simulink model "SimplifiedModelWithRefSearch"  (R2022b)
settings: Solver=VariableStepAuto  StartTime=0.0  StopTime=inf  RelTol=1e-3
model workspace (MAT data in the model file):
  firstWarning = 1
  originalScenarioChecksum = '114339432DE22364D47BB28FC96DC10C'
undefined symbols (not defined in the file): Acceleration, ActorID, AngularVelocity, curvature1, DefaultGear, DEND_B, DEND_S, DEND_T, EgoRefPose, LF, LR, MAX_BRAKE, MAX_STEER, MAX_TORQUE, MCAR, MIN_BRAKE, MIN_STEER, MIN_TORQUE, NUMD_B, NUMD_S, NUMD_T, Pitch, Position, psi_o, R, Roll, RRdamp, session, sigbuilder_block, STEER_RATIO, stopSign_ID, Tdead, TL_ID, TrackWidth, ts, Ts, Vdead, Velocity, X_o, Y_o, Yaw
libraries: drivingvehiclecontroller x2, drivingscenarioandsensors x2, autolibshared x1, vehdynlibviscommon x1, vehdynlibsteering x1
(part 2 of 2)

== matlab function SimplifiedModelWithRefSearch/MATLAB Function ==
  data: RefPose input; RPose output; CurPose input; Curvature output; RefCurve input; j output
function [RPose,Curvature,j] = RefPoseSearch(RefPose,CurPose, RefCurve)

RPose = zeros(1,3);
% RPose = CurPose;
Curvature = 0;
%br = 0;
m = 0; mm = 0; b = 0; bb = 0;
% dth =  5;
% RefPose(:,2:3) = -RefPose(:,2:3);
% CurPose(2:3) = -CurPose(2:3);
dist = zeros(length(RefPose),1);
% a1 =0;a2 =0;a3 =0;a4 =0;

for j = 1:length(RefPose)
    dist(j) = norm(CurPose(1:2) - RefPose(j,1:2));
end

[val,ind] = mink(dist,2);
j = ind(1);

if ind(1) > ind(2)
    ind = [ind(2) ;ind(1)];
end
    
m = (RefPose(ind(1),2) - RefPose(ind(2),2))/(RefPose(ind(1),1) - RefPose(ind(2),1));
if m == inf
    RPose = [RefPose(ind(1),1) CurPose(2) atan2d(RefPose(ind(2),2)-RefPose(ind(2),2),RefPose(ind(2),1)-RefPose(ind(2),1))];
elseif m == 0
    RPose = [CurPose(1) RefPose(ind(1),2) atan2d(RefPose(ind(2),2)-RefPose(ind(2),2),RefPose(ind(2),1)-RefPose(ind(2),1))];
else
    b = RefPose(ind(1),2) - m*RefPose(ind(1),1);
    mm = -1/m;
    bb = CurPose(2) - mm*CurPose(1);
    RPose(1:2) = [(b-bb)/(mm-m) m*((b-bb)/(mm-m))+b]; 
%     RPose(3) = atan2d(-(RefPose(ind(1),2)-RPose(2)),-(RefPose(ind(1),1)-RPose(1))); % RefPose(ind(1),3);
    Curvature = RefCurve(ind(1));
     RPose(3) = RefPose(ind(1),3);

%     RPose(3) = (RefPose(ind(1),3) + RefPose(ind(2),3))/2;
%     Curvature = (RefCurve(ind(1)) + RefCurve(ind(2)))/2;

%     if abs(RefPose(ind(1),3)) < 45 || abs(RefPose(ind(1),3)) > 135
%         Curvature = interp1([RefPose(ind(1),1) RefPose(ind(2),1)],[RefCurve(ind(1)) RefCurve(ind(2))],CurPose(1));
%         RPose(3) = interp1([RefPose(ind(1),1) RefPose(ind(2),1)],[RefPose(ind(1),3) RefPose(ind(2),3)],CurPose(1));
%     else
% %         a1 =RefPose(ind(1),2);a2 =RefPose(ind(2),2);a3 =RefPose(ind(1),3);a4 =RefPose(ind(2),3);
%         Curvature = interp1([RefPose(ind(1),2) RefPose(ind(2),2)],[RefCurve(ind(1)) RefCurve(ind(2))],CurPose(2));
%         RPose(3) = interp1([RefPose(ind(1),2) RefPose(ind(2),2)],[RefPose(ind(1),3) RefPose(ind(2),3)],CurPose(2));
%     end
end



% for j = 1:length(RefPose)-1
%     
%     if (CurPose(3) >= -90 && CurPose(3) <= 90) % Ego vehicle is heading to the "right"
% 
%         if (RefPose(j,3) >= 0 && RefPose(j,3) <= 90) % Positive slope path
%             if RefPose(j,3) > dth && RefPose(j,3) < 90-dth % Ref path is not horizontal nor vertical
% 
%                 if (CurPose(1) >= RefPose(j,1) && CurPose(1) < RefPose(j+1,1)) && (CurPose(2) >= RefPose(j,2) && CurPose(2) < RefPose(j+1,2))
%                     m = (RefPose(j+1,2) - RefPose(j,2))/(RefPose(j+1,1) - RefPose(j,1));
%                     if m == inf
%                         RPose = [RefPose(j,1) CurPose(2) atan2d(RefPose(j+1,2)-RefPose(j,2),RefPose(j+1,1)-RefPose(j,1))];
%                     elseif m == 0
%                         RPose = [CurPose(1) RefPose(j,2) atan2d(RefPose(j+1,2)-RefPose(j,2),RefPose(j+1,1)-RefPose(j,1))];
%                     else
%                         b = RefPose(j,2) - m*RefPose(j,1);
%                         mm = -1/m;
%                         bb = CurPose(2) - mm*CurPose(1);
%                         RPose(1:2) = [(b-bb)/(mm-m) m*((b-bb)/(mm-m))+b];
%                         RPose(3) = interp1([RefPose(j,1) RefPose(j+1,1)],[RefPose(j,3) RefPose(j+1,3)],CurPose(1)); % or atan2d
%                         Curvature = interp1([RefPose(j,1) RefPose(j+1,1)],[RefCurve(j) RefCurve(j+1)],CurPose(1));
%                     end
%                     break;
%                 else
%                     continue
%                 end
% 
%             elseif RefPose(j,3) < dth % Ref path is horizontal
%                 if (CurPose(1) >= RefPose(j,1) && CurPose(1) < RefPose(j+1,1))
%                     m = (RefPose(j+1,2) - RefPose(j,2))/(RefPose(j+1,1) - RefPose(j,1));
%                     if m == inf
%                         RPose = [RefPose(j,1) CurPose(2) atan2d(RefPose(j+1,2)-RefPose(j,2),RefPose(j+1,1)-RefPose(j,1))];
%                     elseif m == 0
%                         RPose = [CurPose(1) RefPose(j,2) atan2d(RefPose(j+1,2)-RefPose(j,2),RefPose(j+1,1)-RefPose(j,1))];
%                     else
%                         b = RefPose(j,2) - m*RefPose(j,1);
%                         mm = -1/m;
%                         bb = CurPose(2) - mm*CurPose(1);
%                         RPose(1:2) = [(b-bb)/(mm-m) m*((b-bb)/(mm-m))+b];
%                         RPose(3) = interp1([RefPose(j,1) RefPose(j+1,1)],[RefPose(j,3) RefPose(j+1,3)],CurPose(1)); % or atan2d
%                         Curvature = interp1([RefPose(j,1) RefPose(j+1,1)],[RefCurve(j) RefCurve(j+1)],CurPose(1));
%                     end
%                     break;
%                 else
%                     continue
%                 end
%             elseif RefPose(j,3) > 90-dth % Ref path is vertical
%                 if (CurPose(2) >= RefPose(j,2) && CurPose(2) < RefPose(j+1,2))
%                     m = (RefPose(j+1,2) - RefPose(j,2))/(RefPose(j+1,1) - RefPose(j,1));
%                     if m == inf
%                         RPose = [RefPose(j,1) CurPose(2) atan2d(RefPose(j+1,2)-RefPose(j,2),RefPose(j+1,1)-RefPose(j,1))];
%                     elseif m == 0
%                         RPose = [CurPose(1) RefPose(j,2) atan2d(RefPose(j+1,2)-RefPose(j,2),RefPose(j+1,1)-RefPose(j,1))];
%                     else
%                         b = RefPose(j,2) - m*RefPose(j,1);
%                         mm = -1/m;
%                         bb = CurPose(2) - mm*CurPose(1);
%                         RPose(1:2) = [(b-bb)/(mm-m) m*((b-bb)/(mm-m))+b];
%                         RPose(3) = interp1([RefPose(j,2) RefPose(j+1,2)],[RefPose(j,3) RefPose(j+1,3)],CurPose(2)); % or atan2d
%                         Curvature = interp1([RefPose(j,2) RefPose(j+1,2)],[RefCurve(j) RefCurve(j+1)],CurPose(2));
%                     end
%                     break;
%                 else
%                     continue
%                 end
%             end
% 
%         elseif (RefPose(j,3) >= -90 && RefPose(j,3) < 0) % Negative slope path
%             if RefPose(j,3) < -dth && RefPose(j,3) > -90+dth % Ref path is not horizontal nor vertical
%                 if (CurPose(1) >= RefPose(j,1) && CurPose(1) < RefPose(j+1,1)) && (CurPose(2) <= RefPose(j,2) && CurPose(2) > RefPose(j+1,2))
%                     m = (RefPose(j+1,2) - RefPose(j,2))/(RefPose(j+1,1) - RefPose(j,1));
%                     if m == inf
%                         RPose = [RefPose(j,1) CurPose(2) atan2d(RefPose(j+1,2)-RefPose(j,2),RefPose(j+1,1)-RefPose(j,1))];
%                     elseif m == 0
%                         RPose = [CurPose(1) RefPose(j,2) atan2d(RefPose(j+1,2)-RefPose(j,2),RefPose(j+1,1)-RefPose(j,1))];
%                     else
%                         b = RefPose(j,2) - m*RefPose(j,1);
%                         mm = -1/m;
%                         bb = CurPose(2) - mm*CurPose(1);
%                         RPose(1:2) = [(b-bb)/(mm-m) m*((b-bb)/(mm-m))+b];
%                         RPose(3) = interp1([RefPose(j,1) RefPose(j+1,1)],[RefPose(j,3) RefPose(j+1,3)],CurPose(1)); % or atan2d
%                         Curvature = interp1([RefPose(j,1) RefPose(j+1,1)],[RefCurve(j) RefCurve(j+1)],CurPose(1));
%                     end
%                     break;
%                 else
%                     continue
%                 end
%             elseif RefPose(j,3) > -dth % Ref path is horizontal
%                 if (CurPose(1) >= RefPose(j,1) && CurPose(1) < RefPose(j+1,1))
%                     m = (RefPose(j+1,2) - RefPose(j,2))/(RefPose(j+1,1) - RefPose(j,1));
%                     if m == inf
%                         RPose = [RefPose(j,1) CurPose(2) atan2d(RefPose(j+1,2)-RefPose(j,2),RefPose(j+1,1)-RefPose(j,1))];
%                     elseif m == 0
%                         RPose = [CurPose(1) RefPose(j,2) atan2d(RefPose(j+1,2)-RefPose(j,2),RefPose(j+1,1)-RefPose(j,1))];
%                     else
%                         b = RefPose(j,2) - m*RefPose(j,1);
%                         mm = -1/m;
%                         bb = CurPose(2) - mm*CurPose(1);
%                         RPose(1:2) = [(b-bb)/(mm-m) m*((b-bb)/(mm-m))+b];
%                         RPose(3) = interp1([RefPose(j,1) RefPose(j+1,1)],[RefPose(j,3) RefPose(j+1,3)],CurPose(1)); % or atan2d
%                         Curvature = interp1([RefPose(j,1) RefPose(j+1,1)],[RefCurve(j) RefCurve(j+1)],CurPose(1));
%                     end
%                     break;
%                 else
%                     continue
%                 end
%             elseif RefPose(j,3) < -90+dth % Ref path is vertical
%                 if (CurPose(2) <= RefPose(j,2) && CurPose(2) > RefPose(j+1,2))
%                     m = (RefPose(j+1,2) - RefPose(j,2))/(RefPose(j+1,1) - RefPose(j,1));
%                     if m == inf
%                         RPose = [RefPose(j,1) CurPose(2) atan2d(RefPose(j+1,2)-RefPose(j,2),RefPose(j+1,1)-RefPose(j,1))];
%                     elseif m == 0
%                         RPose = [CurPose(1) RefPose(j,2) atan2d(RefPose(j+1,2)-RefPose(j,2),RefPose(j+1,1)-RefPose(j,1))];
%                     else
%                         b = RefPose(j,2) - m*RefPose(j,1);
%                         mm = -1/m;
%                         bb = CurPose(2) - mm*CurPose(1);
%                         RPose(1:2) = [(b-bb)/(mm-m) m*((b-bb)/(mm-m))+b];
%                         RPose(3) = interp1([RefPose(j,2) RefPose(j+1,2)],[RefPose(j,3) RefPose(j+1,3)],CurPose(2)); % or atan2d
%                         Curvature = interp1([RefPose(j,2) RefPose(j+1,2)],[RefCurve(j) RefCurve(j+1)],CurPose(2));
%                     end
%                     break;
%                 else
%                     continue
%                 end
%             end
% 
%         else
%             continue
%         end
% 
%     elseif (CurPose(3) > 90 || CurPose(3) < -90) % Ego vehicle is heading to the "left" ("or" is because it does not exceed +-180)
% 
%         if (RefPose(j,3) > 90 && RefPose(j,3) <= 180) % Positive slope path (considering ego vehicle's heading direction)
%             if RefPose(j,3) > 90+dth && RefPose(j,3) < 180-dth % Ref path is not horizontal nor vertical
%                 if (CurPose(1) <= RefPose(j,1) && CurPose(1) > RefPose(j+1,1)) && (CurPose(2) >= RefPose(j,2) && CurPose(2) < RefPose(j+1,2))
%                     m = (RefPose(j+1,2) - RefPose(j,2))/(RefPose(j+1,1) - RefPose(j,1));
%                     if m == inf
%                         RPose = [RefPose(j,1) CurPose(2) atan2d(RefPose(j+1,2)-RefPose(j,2),RefPose(j+1,1)-RefPose(j,1))];
%                     elseif m == 0
%                         RPose = [CurPose(1) RefPose(j,2) atan2d(RefPose(j+1,2)-RefPose(j,2),RefPose(j+1,1)-RefPose(j,1))];
%                     else
%                         b = RefPose(j,2) - m*RefPose(j,1);
%                         mm = -1/m;
%                         bb = CurPose(2) - mm*CurPose(1);
%                         RPose(1:2) = [(b-bb)/(mm-m) m*((b-bb)/(mm-m))+b];
%                         RPose(3) = interp1([RefPose(j,1) RefPose(j+1,1)],[RefPose(j,3) RefPose(j+1,3)],CurPose(1)); % or atan2d
%                         Curvature = interp1([RefPose(j,1) RefPose(j+1,1)],[RefCurve(j) RefCurve(j+1)],CurPose(1));
%                     end
%                     break;
%                 else
%                     continue
%                 end
%             elseif RefPose(j,3) > 180-dth % Ref path is horizontal
%                 if (CurPose(1) <= RefPose(j,1) && CurPose(1) > RefPose(j+1,1))
%                     m = (RefPose(j+1,2) - RefPose(j,2))/(RefPose(j+1,1) - RefPose(j,1));
%                     if m == inf
%                         RPose = [RefPose(j,1) CurPose(2) atan2d(RefPose(j+1,2)-RefPose(j,2),RefPose(j+1,1)-RefPose(j,1))];
%                     elseif m == 0
%                         RPose = [CurPose(1) RefPose(j,2) atan2d(RefPose(j+1,2)-RefPose(j,2),RefPose(j+1,1)-RefPose(j,1))];
%                     else
%                         b = RefPose(j,2) - m*RefPose(j,1);
%                         mm = -1/m;
%                         bb = CurPose(2) - mm*CurPose(1);
%                         RPose(1:2) = [(b-bb)/(mm-m) m*((b-bb)/(mm-m))+b];
%                         RPose(3) = interp1([RefPose(j,1) RefPose(j+1,1)],[RefPose(j,3) RefPose(j+1,3)],CurPose(1)); % or atan2d
%                         Curvature = interp1([RefPose(j,1) RefPose(j+1,1)],[RefCurve(j) RefCurve(j+1)],CurPose(1));
%                     end
%                     break;
%                 else
%                     continue
%                 end
%             elseif RefPose(j,3) < 90+dth % Ref path is vertical
%                 if (CurPose(2) >= RefPose(j,2) && CurPose(2) < RefPose(j+1,2))
%                     m = (RefPose(j+1,2) - RefPose(j,2))/(RefPose(j+1,1) - RefPose(j,1));
%                     if m == inf
%                         RPose = [RefPose(j,1) CurPose(2) atan2d(RefPose(j+1,2)-RefPose(j,2),RefPose(j+1,1)-RefPose(j,1))];
%                     elseif m == 0
%                         RPose = [CurPose(1) RefPose(j,2) atan2d(RefPose(j+1,2)-RefPose(j,2),RefPose(j+1,1)-RefPose(j,1))];
%                     else
%                         b = RefPose(j,2) - m*RefPose(j,1);
%                         mm = -1/m;
%                         bb = CurPose(2) - mm*CurPose(1);
%                         RPose(1:2) = [(b-bb)/(mm-m) m*((b-bb)/(mm-m))+b];
%                         RPose(3) = interp1([RefPose(j,2) RefPose(j+1,2)],[RefPose(j,3) RefPose(j+1,3)],CurPose(2)); % or atan2d
%                         Curvature = interp1([RefPose(j,2) RefPose(j+1,2)],[RefCurve(j) RefCurve(j+1)],CurPose(2));
%                     end
%                     break;
%                 else
%                     continue
%                 end
%             end
% 
%         elseif (RefPose(j,3) > -180 && RefPose(j,3) < -90) % Negative slope path (considering ego vehicle's heading direction)
%             if RefPose(j,3) > -180+dth && RefPose(j,3) < -90-dth % Ref path is not horizontal nor vertical
%                 if (CurPose(1) <= RefPose(j,1) && CurPose(1) > RefPose(j+1,1)) && (CurPose(2) <= RefPose(j,2) && CurPose(2) > RefPose(j+1,2))
%                     m = (RefPose(j+1,2) - RefPose(j,2))/(RefPose(j+1,1) - RefPose(j,1));
%                     if m == inf
%                         RPose = [RefPose(j,1) CurPose(2) atan2d(RefPose(j+1,2)-RefPose(j,2),RefPose(j+1,1)-RefPose(j,1))];
%                     elseif m == 0
%                         RPose = [CurPose(1) RefPose(j,2) atan2d(RefPose(j+1,2)-RefPose(j,2),RefPose(j+1,1)-RefPose(j,1))];
%                     else
%                         b = RefPose(j,2) - m*RefPose(j,1);
%                         mm = -1/m;
%                         bb = CurPose(2) - mm*CurPose(1);
%                         RPose(1:2) = [(b-bb)/(mm-m) m*((b-bb)/(mm-m))+b];
%                         RPose(3) = interp1([RefPose(j,1) RefPose(j+1,1)],[RefPose(j,3) RefPose(j+1,3)],CurPose(1)); % or atan2d
%                         Curvature = interp1([RefPose(j,1) RefPose(j+1,1)],[RefCurve(j) RefCurve(j+1)],CurPose(1));
%                     end
%                     break;
%                 else
%                     continue
%                 end
%             elseif RefPose(j,3) < -180+dth % Ref path is horizontal
%                 if (CurPose(1) <= RefPose(j,1) && CurPose(1) > RefPose(j+1,1))
%                     m = (RefPose(j+1,2) - RefPose(j,2))/(RefPose(j+1,1) - RefPose(j,1));
%                     if m == inf
%                         RPose = [RefPose(j,1) CurPose(2) atan2d(RefPose(j+1,2)-RefPose(j,2),RefPose(j+1,1)-RefPose(j,1))];
%                     elseif m == 0
%                         RPose = [CurPose(1) RefPose(j,2) atan2d(RefPose(j+1,2)-RefPose(j,2),RefPose(j+1,1)-RefPose(j,1))];
%                     else
%                         b = RefPose(j,2) - m*RefPose(j,1);
%                         mm = -1/m;
%                         bb = CurPose(2) - mm*CurPose(1);
%                         RPose(1:2) = [(b-bb)/(mm-m) m*((b-bb)/(mm-m))+b];
%                         RPose(3) = interp1([RefPose(j,1) RefPose(j+1,1)],[RefPose(j,3) RefPose(j+1,3)],CurPose(1)); % or atan2d
%                         Curvature = interp1([RefPose(j,1) RefPose(j+1,1)],[RefCurve(j) RefCurve(j+1)],CurPose(1));
%                     end
%                     break;
%                 else
%                     continue
%                 end
%             elseif RefPose(j,3) > -90-dth % Ref path is vertical
%                 if (CurPose(2) <= RefPose(j,2) && CurPose(2) > RefPose(j+1,2))
%                     m = (RefPose(j+1,2) - RefPose(j,2))/(RefPose(j+1,1) - RefPose(j,1));
%                     if m == inf
%                         RPose = [RefPose(j,1) CurPose(2) atan2d(RefPose(j+1,2)-RefPose(j,2),RefPose(j+1,1)-RefPose(j,1))];
%                     elseif m == 0
%                         RPose = [CurPose(1) RefPose(j,2) atan2d(RefPose(j+1,2)-RefPose(j,2),RefPose(j+1,1)-RefPose(j,1))];
%                     else
%                         b = RefPose(j,2) - m*RefPose(j,1);
%                         mm = -1/m;
%                         bb = CurPose(2) - mm*CurPose(1);
%                         RPose(1:2) = [(b-bb)/(mm-m) m*((b-bb)/(mm-m))+b];
%                         RPose(3) = interp1([RefPose(j,2) RefPose(j+1,2)],[RefPose(j,3) RefPose(j+1,3)],CurPose(2)); % or atan2d
%                         Curvature = interp1([RefPose(j,2) RefPose(j+1,2)],[RefCurve(j) RefCurve(j+1)],CurPose(2));
%                     end
%                     break;
%                 else
%                     continue
%                 end
%             end
%         else
%             continue
%         end
%     end
%      
% end
% RPose(2:3) = -RPose(2:3);






% for j = 1:length(RefPose)-1
%     
%     if CurPose(3) >= 0 && CurPose(3) < 90
%         
%         if (CurPose(1) >= RefPose(j,1) && CurPose(1) < RefPose(j+1,1)) && (CurPose(2) >= RefPose(j,2) && CurPose(2) < RefPose(j+1,2))
%             RPose(2) = interp1([RefPose(j,1) RefPose(j+1,1)],[RefPose(j,2) RefPose(j+1,2)],CurPose(1));
%             RPose(1) = interp1([RefPose(j,2) RefPose(j+1,2)],[RefPose(j,1) RefPose(j+1,1)],CurPose(2));
%             RPose(3) = interp1([RefPose(j,1) RefPose(j+1,1)],[RefPose(j,3) RefPose(j+1,3)],CurPose(1));
%             Curvature = interp1([RefPose(j,1) RefPose(j+1,1)],[RefCurve(j) RefCurve(j+1)],CurPose(1));
%             br = 1; break;
%         else
%             continue
%         end
% 
%     elseif CurPose(3) >= 90 && CurPose(3) <= 180
% 
%         if (CurPose(1) <= RefPose(j,1) && CurPose(1) > RefPose(j+1,1)) && (CurPose(2) >= RefPose(j,2) && CurPose(2) < RefPose(j+1,2))
%             RPose(2) = interp1([RefPose(j,1) RefPose(j+1,1)],[RefPose(j,2) RefPose(j+1,2)],CurPose(1));
%             RPose(1) = interp1([RefPose(j,2) RefPose(j+1,2)],[RefPose(j,1) RefPose(j+1,1)],CurPose(2));
%             RPose(3) = interp1([RefPose(j,1) RefPose(j+1,1)],[RefPose(j,3) RefPose(j+1,3)],CurPose(1));
%             Curvature = interp1([RefPose(j,1) RefPose(j+1,1)],[RefCurve(j) RefCurve(j+1)],CurPose(1));
%             br = 1; break;
%         else
%             continue
%         end
% 
%     elseif CurPose(3) >= -180 && CurPose(3) < -90
% 
%         if (CurPose(1) <= RefPose(j,1) && CurPose(1) > RefPose(j+1,1)) && (CurPose(2) <= RefPose(j,2) && CurPose(2) > RefPose(j+1,2))
%             RPose(2) = interp1([RefPose(j,1) RefPose(j+1,1)],[RefPose(j,2) RefPose(j+1,2)],CurPose(1));
%             RPose(1) = interp1([RefPose(j,2) RefPose(j+1,2)],[RefPose(j,1) RefPose(j+1,1)],CurPose(2));
%             RPose(3) = interp1([RefPose(j,1) RefPose(j+1,1)],[RefPose(j,3) RefPose(j+1,3)],CurPose(1));
%             Curvature = interp1([RefPose(j,1) RefPose(j+1,1)],[RefCurve(j) RefCurve(j+1)],CurPose(1));
%             br = 1; break;
%         else
%             continue
%         end
% 
%     elseif CurPose(3) >= -90 && CurPose(3) < 0
% 
%         if (CurPose(1) >= RefPose(j,1) && CurPose(1) < RefPose(j+1,1)) && (CurPose(2) <= RefPose(j,2) && CurPose(2) > RefPose(j+1,2))
%             RPose(2) = interp1([RefPose(j,1) RefPose(j+1,1)],[RefPose(j,2) RefPose(j+1,2)],CurPose(1));
%             RPose(1) = interp1([RefPose(j,2) RefPose(j+1,2)],[RefPose(j,1) RefPose(j+1,1)],CurPose(2));
%             RPose(3) = interp1([RefPose(j,1) RefPose(j+1,1)],[RefPose(j,3) RefPose(j+1,3)],CurPose(1));
%             Curvature = interp1([RefPose(j,1) RefPose(j+1,1)],[RefCurve(j) RefCurve(j+1)],CurPose(1));
%             br = 1; break;
%         else
%             continue
%         end
% 
%     end
%     
%     if br == 1
%         break;
%     end
% 
% 
% end

== matlab function SimplifiedModelWithRefSearch/Vehicle Dynamics1/Info2ActorState/MATLAB Function ==
  data: X input; Position output; Y input; Z input
function Position = fcn(X, Y, Z)

Position = [X Y, Z];

== matlab function SimplifiedModelWithRefSearch/MATLAB Function1 ==
  settings: updateMethod=DISCRETE
  data: aPose output; Pose input; nPose output; nfactor input
function [aPose,nPose] = noise(Pose,nfactor)

nPose = (1-nfactor + (2*nfactor)*rand)*Pose;
aPose = Pose;

== matlab function SimplifiedModelWithRefSearch/Vehicle Dynamics1/Info2ActorState/MATLAB Function1 ==
  data: Xdot input; Velocity output; Ydot input; Zdot input
function Velocity = fcn(Xdot, Ydot, Zdot)

Velocity = [Xdot Ydot, Zdot];

== matlab function SimplifiedModelWithRefSearch/Vehicle Dynamics1/Info2ActorState/MATLAB Function2 ==
  data: aX input; Acceleration output; aY input; aZ input
function Acceleration = fcn(aX, aY, aZ)

Acceleration = [aX aY, aZ];

== matlab function SimplifiedModelWithRefSearch/Vehicle Dynamics1/Info2ActorState/MATLAB Function3 ==
  data: phiDot input; AngularVelocity output; thetaDot input; psiDot input
function AngularVelocity = fcn(phiDot, thetaDot, psiDot)

AngularVelocity = [phiDot thetaDot, psiDot];

== stateflow chart SimplifiedModelWithRefSearch/Vehicle Dynamics1/VehicleDynamics/engine-steer-brake dynamics/GearSelection1 ==
  state Park
    CurrGear = 0;
  state Reverse
    CurrGear = -1;
  state drive
    CurrGear = 1;
  (default) -> (junction 12)
  (junction 12) -> Reverse [order 3] : [DefaultGear == -1]
  (junction 12) -> drive [order 2] : [DefaultGear == 1]
  (junction 12) -> Park [order 1] : [DefaultGear == 0]
  (junction 12) -> Park [order 4] : %fallback to park
  drive -> Park [order 2] : [gear_cmd == 0 && allowShift(vc,Tbrake)]
  Park -> Reverse [order 2] : [gear_cmd == -1 && allowShift(vc,Tbrake)]
  Park -> drive [order 1] : [gear_cmd == 1 && allowShift(vc,Tbrake)]
  Reverse -> Park [order 2] : [gear_cmd == 0 && allowShift(vc,Tbrake)]
  drive -> Reverse [order 1] : [gear_cmd == -1 && allowShift(vc,Tbrake)]
  Reverse -> drive [order 1] : [gear_cmd == 1 && allowShift(vc,Tbrake)]
  data: Tdead parameter; Vdead parameter; vel function_input; brakeT function_input; allow function_output; CurrGear output; Tbrake input; vc input; gear_cmd input; DefaultGear parameter
  function allow = allowShift(vel, brakeT):
    | function allow = allowShift(vel, brakeT)
    | allow = (abs(vel) <= Vdead) && (abs(brakeT)>Tdead);
    | end

== matlab function SimplifiedModelWithRefSearch/Vehicle Dynamics1/VehicleDynamics/engine-steer-brake dynamics/compute net torque ==
  data: gear input; Tnet output; Tengine input; Tbrake input; vc input
function Tnet  = net_torque(gear,Tengine,Tbrake,vc)

%  --set engine torque based on current gear selection

if (gear == 0)
    %  --vehicle is in PARK, so force engine torque to zero
    Tengine = 0;
end

Tnet = Tengine + Tbrake*tanh(5*vc);

end

== matlab function SimplifiedModelWithRefSearch/Vehicle Dynamics1/VehicleDynamics/engine-steer-brake dynamics/gear selection state machine ==
  data: gear output; gear_cmd input; vc input; Tbrake input; Tdead input; Vdead input
function gear = gear_change_FSM(gear_cmd,vc,Tbrake,Tdead,Vdead)

persistent GEAR

%  The vehicle gear can take on one of the following enumerated values:
%  -1 = REVERSE
%   0 = PARK
%   1 = DRIVE

%  --initialize the local persistent variables

if isempty(GEAR)
    %  --default gear at startup is PARK
    %  Note:  Change this to 1 if you want car to initialize in DRIVE
    GEAR = 0;
end


%  --evaluate the gear change finite state machine

switch GEAR
    case 0  % vehicle is in PARK
        if (gear_cmd == 1)
            %  --check to see if we can shift to DRIVE
            if ((abs(vc) <= Vdead) && (abs(Tbrake) > Tdead))
                %  --shift to DRIVE
                GEAR = 1;
            end
            
        elseif (gear_cmd == 2)
            %  --check to see if we can shift to REVERSE
            if ((abs(vc) <= Vdead) && (abs(Tbrake) > Tdead))
                %  --shift to REVERSE
                GEAR = 2;
            end
        end
        
    case 1  % vehicle is in DRIVE
        if (gear_cmd == 0)
            %  --check to see if we can shift to PARK
            if ((abs(vc) <= Vdead) && (abs(Tbrake) > Tdead))
                %  --shift to PARK
                GEAR = 0;
            end
            
        elseif (gear_cmd == 2)
            %  --check to see if we can shift to REVERSE
            if ((abs(vc) <= Vdead) && (abs(Tbrake) > Tdead))
                %  --shift to REVERSE
                GEAR = 2;
            end
        end
        
    case -1  % vehicle is in REVERSE
        if (gear_cmd == 0)
            %  --check to see if we can shift to PARK
            if ((abs(vc) <= Vdead) && (abs(Tbrake) > Tdead))
                %  --shift to PARK
                GEAR = 0;
            end
            
        elseif (gear_cmd == 1)
            %  --check to see if we can shift to DRIVE
            if ((abs(vc) <= Vdead) && (abs(Tbrake) > Tdead))
                %  --shift to DRIVE
                GEAR = 1;
            end
        end
        
    otherwise  %  --should never be here
        if (vc > Vdead)
            %  --moving forward, so must be in DRIVE
            GEAR = 1;
        elseif (vc < -Vdead)
            %  --moving backward, so must be in REVERSE
            GEAR = 2;
        else
            %  --vehicle stoppped, so must be in PARK
            GEAR = 0;
        end

end


%  --output the current actual gear setting

gear = GEAR;

return

== matlab function SimplifiedModelWithRefSearch/Visualization/Positions and States /MATLAB Function2 ==
  data: Actors input; ss_poses output; ss_State input

function ss_poses = findssposes(Actors, ss_State)

n=length(ss_State);
ss_poses=zeros(n,4);
indices=zeros(n,1);
ID=zeros(length(Actors),1);

for i=1:length(Actors)
 ID(i)=Actors(i).ActorID;
end

indices=find(ismember(ID,ss_State));
if(~isempty(indices))
    
    for i=1:n
        ss_poses(i,:)=([Actors(indices(i)).Position(:)',ss_State(i)]);
    end
end

ss_poses(ss_poses==0)=NaN;






% ss1_poses=zeros(1,4);
% ss2_poses=zeros(1,4);
% for i=1:length(Actors)
%     ID=Actors(i).ActorID;
%     
%     if(ID==ss1_State(1))
%         ss1_poses=[Actors(i).Position(:)',ss1_State(1)];
%     elseif ID== (ss1_State(2))
%         ss2_poses=[Actors(i).Position(:)',ss1_State(2)];
%     
%     end
%   
% end
% ss1_poses(ss1_poses==0)=NaN;   
% ss2_poses(ss2_poses==0)=NaN;

== matlab function SimplifiedModelWithRefSearch/Visualization/Positions and States /MATLAB Function1 ==
  data: Actors input; TL_poses output; TL_State input

function TL_poses = findTLposes(Actors, TL_State)
n=length(TL_State);
TL_poses=zeros(n/2,5);
indices=zeros(n/2,1);
ID=zeros(length(Actors),1);

for i=1:length(Actors)
 ID(i)=Actors(i).ActorID;
end

indices=find(ismember(ID,TL_State(n/2+1:end)));
if (~isempty(indices))

    for i=1:n/2
        TL_poses(i,:)=([Actors(indices(i)).Position(:)',TL_State(i),ID(indices(i))]);

    end
end
TL_poses(TL_poses==0)=NaN;

== stateflow chart SimplifiedModelWithRefSearch/Visualization/Positions and States /Traffic Light Sensor/Traffic Light Switching Logic ==
  state STEADYRED
    entry:
    trafficLight(:)= Red; TL_ID=TL_id;
  state STEADYGREEN
    entry:
    trafficLight(:)= Green; TL_ID=TL_id;
  state START
    entry:
    trafficLight=TL_id;
    trafficLight(:)= Black;TL_ID=TL_id;
  state TRAFFICLIGHT_ODDYELLOW_EVENRED
    entry:
    trafficLight(1:2:end)=Yellow;TL_ID(1:2:end)=TL_id(1:2:end);
    trafficLight(2:2:end) = Red;TL_ID(2:2:end)=TL_id(2:2:end);
  state TRAFFICLIGHT_ODDGREEN_EVENRED
    entry:
    trafficLight(1:2:end)=Green;TL_ID(1:2:end)=TL_id(1:2:end);
    trafficLight(2:2:end) = Red;TL_ID(2:2:end)=TL_id(2:2:end);
  state TRAFFICLIGHT_ODDRED_EVENYELLOW
    entry:
    trafficLight(1:2:end)=Red;TL_ID(1:2:end)=TL_id(1:2:end);
    trafficLight(2:2:end) = Yellow;TL_ID(2:2:end)=TL_id(2:2:end);
  state TRAFFICLIGHT_ODDRED_EVENGREEN
    entry:
    trafficLight(1:2:end)=Red;TL_ID(1:2:end)=TL_id(1:2:end);
    trafficLight(2:2:end) = Green;TL_ID(2:2:end)=TL_id(2:2:end);
  (default) -> START
  START -> STEADYGREEN [order 3] : [LightConfig==1]
  START -> STEADYRED [order 1] : [LightConfig==2]
  START -> TRAFFICLIGHT_ODDGREEN_EVENRED [order 2] : [LightConfig ==3]
  TRAFFICLIGHT_ODDGREEN_EVENRED -> TRAFFICLIGHT_ODDYELLOW_EVENRED : after(4,sec)
  TRAFFICLIGHT_ODDYELLOW_EVENRED -> TRAFFICLIGHT_ODDRED_EVENGREEN : after(1,sec)
  TRAFFICLIGHT_ODDRED_EVENYELLOW -> TRAFFICLIGHT_ODDGREEN_EVENRED : after(1,sec)
  TRAFFICLIGHT_ODDRED_EVENGREEN -> TRAFFICLIGHT_ODDRED_EVENYELLOW : after(4,sec)
  data: Green constant double =3; Red constant double =1; Yellow constant double =2; LightConfig input; TL_id input; Black constant double =0; TL_ID output; trafficLight output
